simulink model "Rollover_Driver"  (R2017a)
settings: Solver=ode45  StartTime=0  StopTime=inf  FixedStep=0.002  RelTol=1e-3  AbsTol=1e-6
values from neighbouring files (symbols this model uses):
  T = [tspan(1):sampling_step_size:tspan(2)]'    [rollover_sim.m]    (also in simulink_test.m = [tspan(1): 0.01: tspan(2)]')
  u_SW = cst_input_init.*zeros(size(T))    [rollover_sim.m]
libraries: Solver_SF x1
settings Model: ExtModeTrigMode=oneshot  ExtModeArmWhenConnect=off  Creator=dhall  LastModifiedBy=Tangsun
settings DataIOCC: SaveFormat=Array  SignalLoggingSaveFormat=ModelDataLogs  SignalLoggingName=sigsOut
settings OptimizationCC: BooleanDataType=off  InitFltsAndDblsToZero=on  LifeSpan=inf
settings DebuggingCC: SaveWithParameterizedLinksMsg=none  UnderspecifiedInitializationDetection=Classic  MergeDetectMultiDrivingBlocksExec=none  SignalResolutionControl=TryResolveAllWithWarning  MultiTaskDSMMsg=warning  MultiTaskCondExecSysMsg=none  FcnCallInpInsideContextMsg=warning  StateNameClashWarn=warning  SFUnexpectedBacktrackingDiag=warning  SFNoUnconditionalDefaultTransitionDiag=warning  SFExecutionAtInitializationDiag=none
settings HardwareCC: ProdBitPerPointer=32  ProdBitPerSizeT=32  ProdBitPerPtrDiffT=32  ProdLargestAtomicFloat=None  ProdIntDivRoundTo=Undefined  ProdEndianess=Unspecified  ProdWordSize=32  ProdHWDeviceType=32-bit Generic  TargetUnknown=on
settings ModelReferenceCC: PropagateSignalLabelsOutOfModel=off
settings RTWCC: TemplateMakefile=grt_vc.tmf
settings GRTTargetCC: TargetFcnLib=ansi_tfl_tmw.mat  TargetLangStandard=C89/C90 (ANSI)  ModelReferenceCompliant=off  CombineOutputUpdateFcns=off  MatFileLogging=off  GRTInterface=on
settings ConfigComp: CovMetricSettings=dw  CovHtmlReporting=on  CovSaveCumulativeToWorkspaceVar=on  CovSaveSingleToWorkspaceVar=on  CovExternalEMLEnable=off

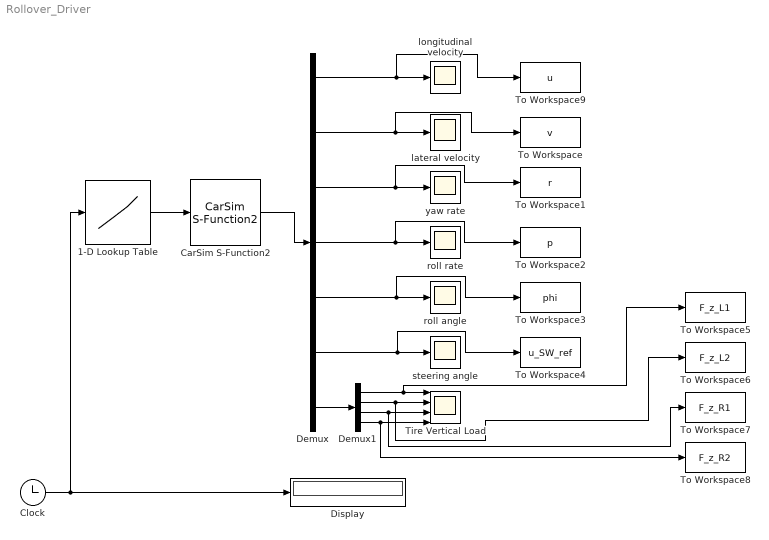
== system Rollover_Driver ==
  1-D Lookup Table : Lookup_n-D  NumberOfTableDimensions=1  BreakpointsForDimension1=T  Table=u_SW  InternalRulePriority=Speed  RndMeth=Simplest  InputSameDT=on
  CarSim S-Function2 : Solver_SF/CarSim S-Function2  Priority=1  VehicleCode=i_i  SIMFILE=simfile.sim
      settings: AttributesFormatString=Vehicle Code: %<VehicleCode>
  Clock : Clock
  Demux : Demux  Outputs=[1 1 1 1 1 1 4]
  Demux1 : Demux
  Display : Display
      settings: Format=bank  Decimation=100
  Tire Vertical Load : Scope  NumInputPorts=4
  To Workspace : ToWorkspace  VariableName=v  SaveFormat=Timeseries  SampleTime=-1
  To Workspace1 : ToWorkspace  VariableName=r  SaveFormat=Timeseries  SampleTime=-1
  To Workspace2 : ToWorkspace  VariableName=p  SaveFormat=Timeseries  SampleTime=-1
  To Workspace3 : ToWorkspace  VariableName=phi  SaveFormat=Timeseries  SampleTime=-1
  To Workspace4 : ToWorkspace  VariableName=u_SW_ref  SaveFormat=Timeseries  SampleTime=-1
  To Workspace5 : ToWorkspace  VariableName=F_z_L1  SaveFormat=Timeseries  SampleTime=-1
  To Workspace6 : ToWorkspace  VariableName=F_z_L2  SaveFormat=Timeseries  SampleTime=-1
  To Workspace7 : ToWorkspace  VariableName=F_z_R1  SaveFormat=Timeseries  SampleTime=-1
  To Workspace8 : ToWorkspace  VariableName=F_z_R2  SaveFormat=Timeseries  SampleTime=-1
  To Workspace9 : ToWorkspace  VariableName=u  SaveFormat=Timeseries  SampleTime=-1
  lateral velocity : Scope
  longitudinal velocity : Scope
  roll angle : Scope
  roll rate : Scope
  "steering angle " : Scope
  yaw rate : Scope
  wires:
  CarSim S-Function2/1 -> Demux/1
  Demux1/1 -> To Workspace5/1, Tire Vertical Load/1
  Demux1/2 -> Tire Vertical Load/2, To Workspace6/1
  Demux1/3 -> To Workspace7/1, Tire Vertical Load/3
  Demux1/4 -> To Workspace8/1, Tire Vertical Load/4
  1-D Lookup Table/1 -> CarSim S-Function2/1
  Clock/1 -> 1-D Lookup Table/1, Display/1
  Demux/7 -> Demux1/1
  Demux/2 -> To Workspace/1, lateral velocity/1
  Demux/3 -> To Workspace1/1, yaw rate/1
  Demux/4 -> To Workspace2/1, roll rate/1
  Demux/5 -> To Workspace3/1, roll angle/1
  Demux/6 -> To Workspace4/1, "steering angle "/1
  Demux/1 -> To Workspace9/1, longitudinal velocity/1
